simulink model "BMS2"  (R2024a)
settings: Solver=VariableStepAuto  StartTime=0.0  StopTime=3600  RelTol=1e-3
undefined symbols (not defined in the file): Ion, Lithium
libraries: spsMosfetLib x9, spsSeriesRLCBranchLib x9, spsBatteryLib x8, spsVoltageMeasurementLib x1, spsControlledCurrentSourceLib x1, spsDCVoltageSourceLib x1, spsDiodeLib x1, spsIdealSwitchLib x1, sps_lib x1
settings Model: Creator=kanna  LastModifiedBy=kanna

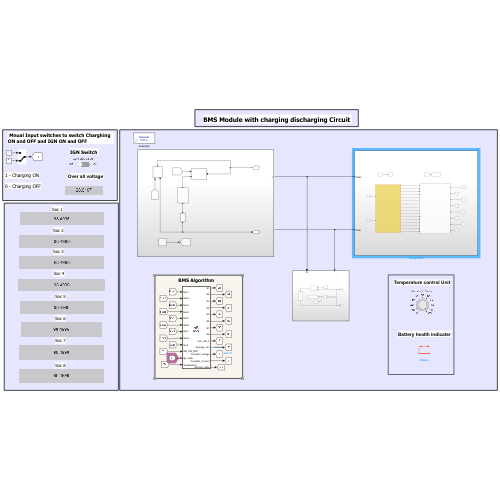
[thumbnail: Simulink's stored preview of the top-level diagram]
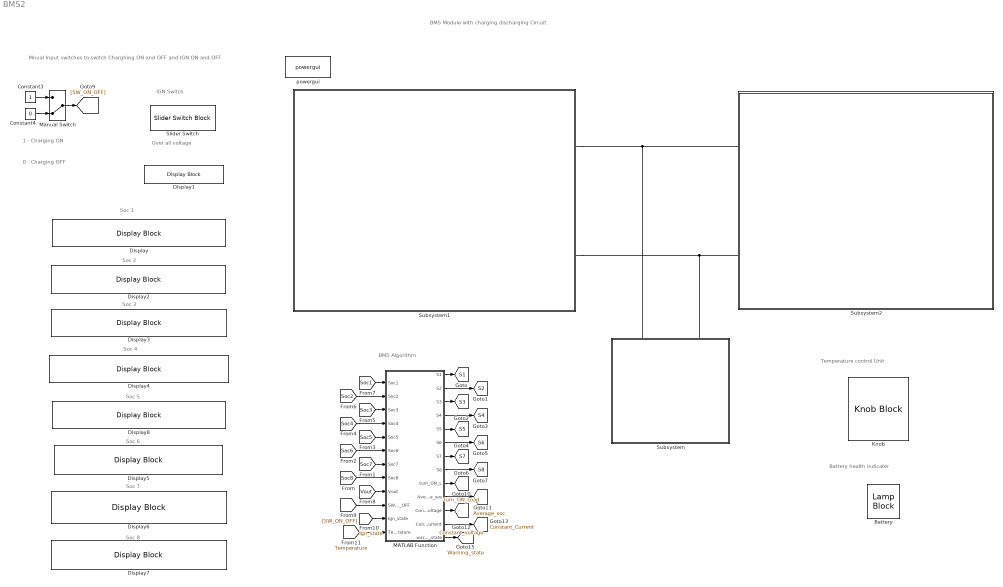
== system BMS2 ==
  note: Over all voltage
  note: Battery health indicater
  note: Temperature control Unit
  note: IGN Switch
  note: Soc 1
  note: 0 - Charging OFF
  note: 1 - Charging ON
  note: Mnual Input switches to switch Charghing ON and OFF and IGN ON and OFF
  note: BMS Algorithm
  note: BMS Module with charging discharging Circuit
  note: Soc 2
  note: Soc 3
  note: Soc 4
  note: Soc 5
  note: Soc 6
  note: Soc 7
  note: Soc 8
  Battery : LampBlock  LabelPosition=Hide  Icon=Battery
  Constant3 : Constant
  Constant4 : Constant  Value=0
  Display{,1..8} (9 alike) : DisplayBlock  LabelPosition=Hide  Transparency=1
  Knob : KnobBlock
  MATLAB Function : MATLAB Function  TreatAsAtomicUnit=on
  Manual Switch : ManualSwitch  CurrentSetting=0
  Slider Switch : SliderSwitchBlock
      settings: Values={{'Off', 'On'}, [0 1]}
  Subsystem : Subsystem
  Subsystem1 : Subsystem
  Subsystem2 : Subsystem
  powergui : sps_lib/powergui  Priority=1  SimulationMode=Discrete  SampleTime=10000e-6  frequency=60  Iterations=50  frequencyindice=0  Pbase=100e6  ErrMax=1e-4  UnitsV=kV  UnitsW=MW  buscounter=0  FunctionMessages=off  echomessages=off  EnableUseOfTLC=off  CurrentSourceSwitches=off  DisableSnubberDevices=off  DisableRonSwitches=off  DisableVfSwitches=off  DisplayEquations=off  AutomaticDiscreteSolvers=off  SolverType=Tustin/Backward Euler (TBE)  Interpol=off  ExternalGateDelay=off  methode=off  Ts=100  x0status=blocks  SPID=on  SwTol=0  HookPort=off  NonlinearTolerance=1e-4  nMaxIteration=100  ContinueOnMaxIteration=off  RestoreLinks=warning  ResistiveCurrentMeasurement=off  Frange=[0:2:500]  Ylog=off  Xlog=on  ShowGrid=off  save=off  variable=ZData  structure=0  ZoomFFT=off  StartTime=0.0  cycles=1  DisplayStyle=1  fundamental=60  FreqAxis=off  MaxFrequency=1000  frequencyindicesteady=1  RmsSteady=1  display=off
  tag scope: Average_soc=global, Constant_Current=global, Constant_voltage=global, S1=global, S2=global, S3=global, S4=global, S5=global, S6=global, S7=global, S8=global, Warning_state=global, turn_ON_Load=global
  wires:
  [Soc1] -> MATLAB Function/1(Soc1)
  [Soc2] -> MATLAB Function/2(Soc2)
  [Soc3] -> MATLAB Function/3(Soc3)
  [Soc4] -> MATLAB Function/4(Soc4)
  [Soc5] -> MATLAB Function/5(Soc5)
  [Soc6] -> MATLAB Function/6(Soc6)
  [Soc7] -> MATLAB Function/7(Soc7)
  [Soc8] -> MATLAB Function/8(Soc8)
  MATLAB Function/1(S1) -> [S1]
  MATLAB Function/5(S5) -> [S5]
  MATLAB Function/2(S2) -> [S2]
  MATLAB Function/3(S3) -> [S3]
  MATLAB Function/4(S4) -> [S4]
  MATLAB Function/6(S6) -> [S6]
  MATLAB Function/7(S7) -> [S7]
  MATLAB Function/8(S8) -> [S8]
  [Vout] -> MATLAB Function/9(Vout)
  Constant3/1 -> Manual Switch/1
  Constant4/1 -> Manual Switch/2
  Manual Switch/1 -> [SW_ON_OFF]
  [SW_ON_OFF] -> MATLAB Function/10(SW_ON_OFF)
  MATLAB Function/9(turn_ON_L) -> [turn_ON_Load]
  MATLAB Function/10(Average_soc) -> [Average_soc]
  MATLAB Function/11(Constant_voltage) -> [Constant_voltage]
  MATLAB Function/12(Constant_Current) -> [Constant_Current]
  [Ign_state] -> MATLAB Function/11(Ign_state)
  [Temperature] -> MATLAB Function/12(Temperature)
  MATLAB Function/13(warning_state) -> [Warning_state]
  connections:
  Subsystem1/RConn1 -- Subsystem2/LConn1 -- Subsystem/LConn1
  Subsystem1/RConn2 -- Subsystem2/LConn2 -- Subsystem/LConn2

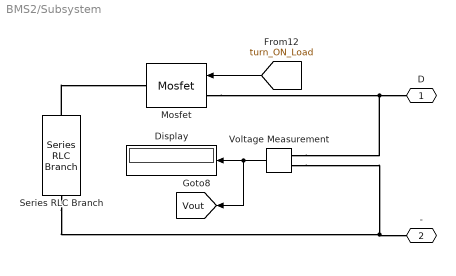
== system BMS2/Subsystem ==
  Display : Display
  Mosfet : spsMosfetLib/Mosfet  Ron=0.1  Lon=0  Rd=0.01  Vfd=0  IC=0  Rs=1e5  Cs=inf  Measurements=off
  Series RLC Branch : spsSeriesRLCBranchLib/Series RLC Branch  LConnTagsString=__new0  RConnTagsString=__new0  BranchType=R  Resistance=50  Inductance=1e-3  SetiL0=off  InitialCurrent=0  Capacitance=1e-6  Setx0=off  InitialVoltage=0  Measurements=None
  Voltage Measurement : spsVoltageMeasurementLib/Voltage Measurement  PhasorSimulation=off  OutputType=Complex  PSBequivalent=0
  D : PMIOPort  Side=Left
  - : PMIOPort  Port=2  Side=Left
  tag scope: Vout=global
  wires:
  [turn_ON_Load] -> Mosfet/1
  Voltage Measurement/1 -> [Vout], Display/1
  connections:
  Series RLC Branch/LConn1 -- Mosfet/RConn1
  Voltage Measurement/LConn1 -- Mosfet/LConn1 -- D/RConn1
  Series RLC Branch/RConn1 -- Voltage Measurement/LConn2 -- -/RConn1

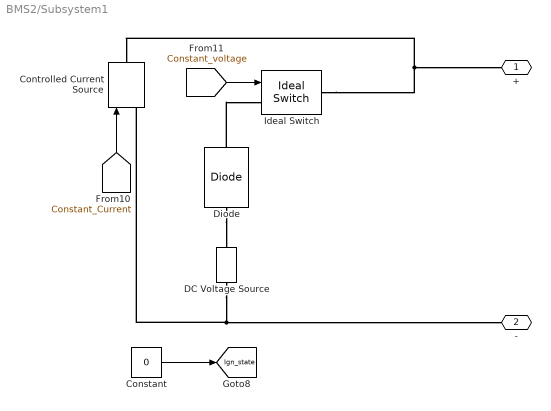
== system BMS2/Subsystem1 ==
  Constant : Constant  Value=0
  Controlled Current Source : spsControlledCurrentSourceLib/Controlled Current Source  Initialize=on  Source_Type=DC  Amplitude=2  Phase=0  Frequency=0  Measurements=None
  DC Voltage Source : spsDCVoltageSourceLib/DC Voltage Source  Amplitude=35  Measurements=None
  Diode : spsDiodeLib/Diode  Ron=0.001  Lon=0  Vf=0.8  IC=0  UseSnubber=0  Rs=500  Cs=250e-9  Measurements=off
  Ideal Switch : spsIdealSwitchLib/Ideal Switch  Ron=0.001  Lon=0  IC=0  Rs=1e5  Cs=inf  Measurements=off
  + : PMIOPort  Side=Right
  - : PMIOPort  Port=2  Side=Right
  tag scope: Ign_state=global
  wires:
  [Constant_voltage] -> Ideal Switch/1
  [Constant_Current] -> Controlled Current Source/1
  Constant/1 -> [Ign_state]
  connections:
  Ideal Switch/RConn1 -- +/RConn1 -- Controlled Current Source/RConn1
  Diode/RConn1 -- Ideal Switch/LConn1
  Diode/LConn1 -- DC Voltage Source/RConn1
  DC Voltage Source/LConn1 -- -/RConn1 -- Controlled Current Source/LConn1

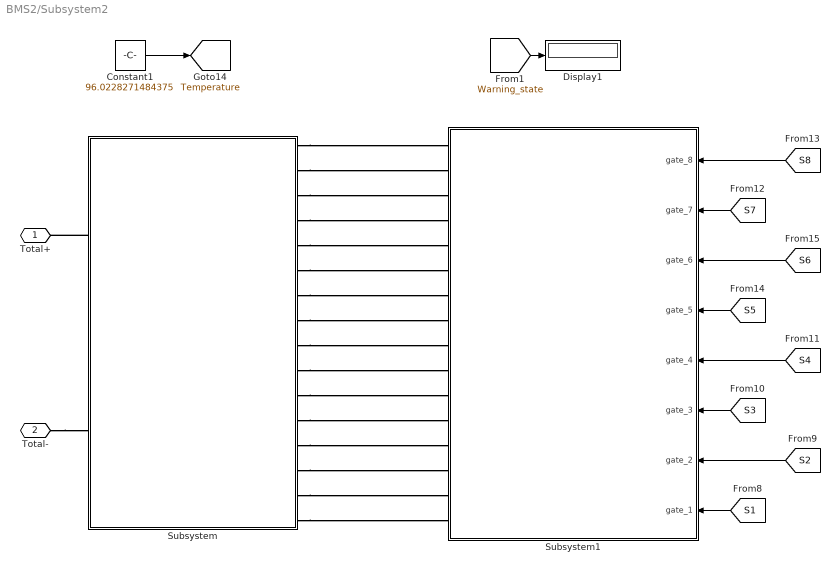
== system BMS2/Subsystem2 ==
  Constant1 : Constant  Value=96.0228271484375
  Display1 : Display
  Subsystem : Subsystem
  Subsystem1 : Subsystem
      settings: PortSchema="{\"entries\":[{\"content\":{\"sides\":[{\"content\":{\"connectorIds\":[\"LConn1\",\"LConn2\",\"LConn3\",\"LConn4\",\"LConn5\",\"LConn6\",\"LConn7\",\"LConn8\",\"LConn9\",\"LConn10\",\"LConn11\",\"LConn12\",\"LConn13\",\"LConn14\",\"LConn15\",\"LConn16\"]},\"type\":\"ConnectorPlacement.EquallySpacedRectSide\",\"uuid\":\"299ba52d-8015-465c-9de8-ad4a2af20b1b\"},{\"content\":{\"connectorIds\":[\"In1\",\"In2\",\"In3\",\"In4\",\"In5\",\"In6\",\"In7\",\"In8\"],\"side\":\"RIGHT\"},\"type\":\"ConnectorPlacement.EquallySpacedRectSide\",\"uuid\":\"0c259d42-c7d5-4490-aca3-04d7e6d01d9f\"},{\"content\":{\"side\":\"TOP\"},\"type\":\"ConnectorPlacement.EquallySpacedRectSide\",\"uuid\":\"1f9aba9e-79c3-4f87-9285-0c028554fb61\"}]},\"type\":\"ConnectorPlacement.EquallySpacedConnector\",\"uuid\":\"3efdec2a-ca98-432c-aa70-a3544e884ae7\"}],\"packageUris\":[\"http://schema.mathworks.com/mf0/Connector/R2020b\"],\"version\":\"1.0\"}"
  Total+ : PMIOPort  Side=Left
  Total- : PMIOPort  Port=2  Side=Left
  tag scope: Temperature=global
  wires:
  [S1] -> Subsystem1/8(gate_1)
  [S4] -> Subsystem1/5(gate_4)
  [S8] -> Subsystem1/1(gate_8)
  [S3] -> Subsystem1/6(gate_3)
  [S7] -> Subsystem1/2(gate_7)
  [S6] -> Subsystem1/3(gate_6)
  [S5] -> Subsystem1/4(gate_5)
  [S2] -> Subsystem1/7(gate_2)
  [Warning_state] -> Display1/1
  Constant1/1 -> [Temperature]
  connections:
  Subsystem/RConn11 -- Subsystem1/LConn11
  Subsystem/RConn2 -- Subsystem1/LConn2
  Subsystem/RConn8 -- Subsystem1/LConn8
  Subsystem/RConn9 -- Subsystem1/LConn9
  Subsystem/RConn5 -- Subsystem1/LConn5
  Total-/RConn1 -- Subsystem/LConn2
  Subsystem/LConn1 -- Total+/RConn1
  Subsystem/RConn3 -- Subsystem1/LConn3
  Subsystem/RConn7 -- Subsystem1/LConn7
  Subsystem/RConn4 -- Subsystem1/LConn4
  Subsystem/RConn1 -- Subsystem1/LConn1
  Subsystem/RConn16 -- Subsystem1/LConn16
  Subsystem/RConn6 -- Subsystem1/LConn6
  Subsystem/RConn12 -- Subsystem1/LConn12
  Subsystem/RConn14 -- Subsystem1/LConn14
  Subsystem/RConn10 -- Subsystem1/LConn10
  Subsystem/RConn13 -- Subsystem1/LConn13
  Subsystem/RConn15 -- Subsystem1/LConn15

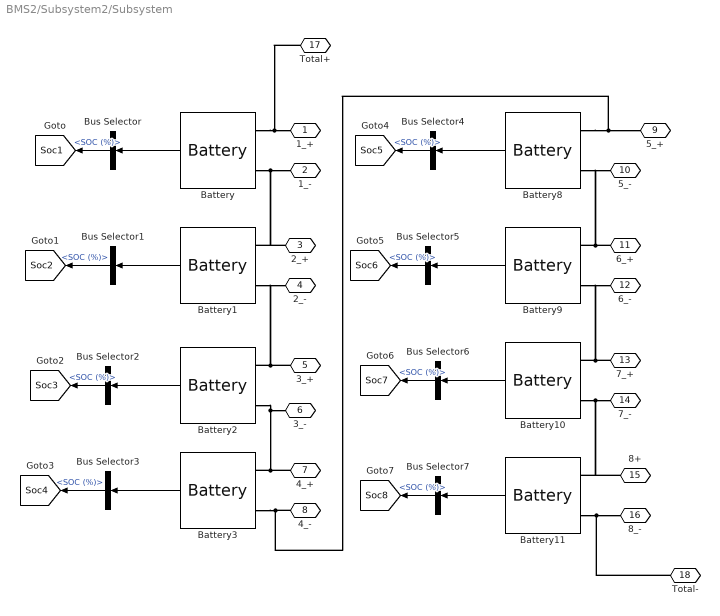
== system BMS2/Subsystem2/Subsystem ==
  Battery : spsBatteryLib/Battery  BatType=Lithium-Ion  ShowTempParam=off  ThermalPreset=no  ShowAgeParam=off  NomV=3.2  NomQ=18  SOC=98.5  Batt_Tr=30  PresetModel=on  MaxQ=18  MinV=2.4  FullV=3.7248  Dis_rate=7.8261  R=0.0017778  Normal_OP=16.2783  expZone="[3.4572     0.88435]"  current=[6.5 13 32.5]  Units=Time  Tci=20  NomT=20  T2=-30  MaxQ2=4.8  FullV2=7.1  Normal_OP2=5.655  expZone2="[6.58           1]"  Rca=0.6  ti=2000  Dp=0  Neq0=0  Tsim=1e6  Ta1=25  Qeol=5.4*0.9  Reol=0.013333*1.2  Char_age=[2.3478, 3]  Dis_age=[2.3478, 10]  N1=1500  N2=10500  N3=1000  N4=1400  Ta2=45  N5=950
  Battery1 : spsBatteryLib/Battery  BatType=Lithium-Ion  ShowTempParam=off  ThermalPreset=no  ShowAgeParam=off  NomV=3.2  NomQ=18  SOC=99  Batt_Tr=30  PresetModel=on  MaxQ=18  MinV=2.4  FullV=3.7248  Dis_rate=7.8261  R=0.0017778  Normal_OP=16.2783  expZone="[3.4572     0.88435]"  current=[6.5 13 32.5]  Units=Time  Tci=20  NomT=20  T2=-30  MaxQ2=4.8  FullV2=7.1  Normal_OP2=5.655  expZone2="[6.58           1]"  Rca=0.6  ti=2000  Dp=0  Neq0=0  Tsim=1e6  Ta1=25  Qeol=5.4*0.9  Reol=0.013333*1.2  Char_age=[2.3478, 3]  Dis_age=[2.3478, 10]  N1=1500  N2=10500  N3=1000  N4=1400  Ta2=45  N5=950
  Battery{2..3,8..11} (6 alike) : spsBatteryLib/Battery  BatType=Lithium-Ion  ShowTempParam=off  ThermalPreset=no  ShowAgeParam=off  NomV=3.2  NomQ=18  SOC=100  Batt_Tr=30  PresetModel=on  MaxQ=18  MinV=2.4  FullV=3.7248  Dis_rate=7.8261  R=0.0017778  Normal_OP=16.2783  expZone="[3.4572     0.88435]"  current=[6.5 13 32.5]  Units=Time  Tci=20  NomT=20  T2=-30  MaxQ2=4.8  FullV2=7.1  Normal_OP2=5.655  expZone2="[6.58           1]"  Rca=0.6  ti=2000  Dp=0  Neq0=0  Tsim=1e6  Ta1=25  Qeol=5.4*0.9  Reol=0.013333*1.2  Char_age=[2.3478, 3]  Dis_age=[2.3478, 10]  N1=1500  N2=10500  N3=1000  N4=1400  Ta2=45  N5=950
  Bus Selector{,1..7} (8 alike) : BusSelector  OutputSignals=SOC (%)
  1_+ : PMIOPort  Side=Right
  1_- : PMIOPort  Port=2  Side=Right
  2_+ : PMIOPort  Port=3  Side=Right
  2_- : PMIOPort  Port=4  Side=Right
  3_+ : PMIOPort  Port=5  Side=Right
  3_- : PMIOPort  Port=6  Side=Right
  4_+ : PMIOPort  Port=7  Side=Right
  4_- : PMIOPort  Port=8  Side=Right
  5_+ : PMIOPort  Port=9  Side=Right
  5_- : PMIOPort  Port=10  Side=Right
  6_+ : PMIOPort  Port=11  Side=Right
  6_- : PMIOPort  Port=12  Side=Right
  7_+ : PMIOPort  Port=13  Side=Right
  7_- : PMIOPort  Port=14  Side=Right
  8+ : PMIOPort  Port=15  Side=Right
  8_- : PMIOPort  Port=16  Side=Right
  Total+ : PMIOPort  Port=17  Side=Left
  Total- : PMIOPort  Port=18  Side=Left
  tag scope: Soc1=global, Soc2=global, Soc3=global, Soc4=global, Soc5=global, Soc6=global, Soc7=global, Soc8=global
  wires:
  Battery1/1 -> Bus Selector1/1
  Bus Selector/1 -> [Soc1]  "<SOC (%)>"
  Battery/1 -> Bus Selector/1
  Bus Selector7/1 -> [Soc8]  "<SOC (%)>"
  Bus Selector5/1 -> [Soc6]  "<SOC (%)>"
  Battery2/1 -> Bus Selector2/1
  Battery11/1 -> Bus Selector7/1
  Bus Selector4/1 -> [Soc5]  "<SOC (%)>"
  Bus Selector6/1 -> [Soc7]  "<SOC (%)>"
  Battery3/1 -> Bus Selector3/1
  Bus Selector3/1 -> [Soc4]  "<SOC (%)>"
  Bus Selector2/1 -> [Soc3]  "<SOC (%)>"
  Bus Selector1/1 -> [Soc2]  "<SOC (%)>"
  Battery8/1 -> Bus Selector4/1
  Battery10/1 -> Bus Selector6/1
  Battery9/1 -> Bus Selector5/1
  connections:
  Battery11/LConn2 -- 8_-/RConn1 -- Total-/RConn1
  3_+/RConn1 -- Battery2/LConn1 -- Battery1/LConn2 -- 2_-/RConn1
  3_-/RConn1 -- Battery2/LConn2 -- 4_+/RConn1 -- Battery3/LConn1
  7_+/RConn1 -- Battery10/LConn1 -- Battery9/LConn2 -- 6_-/RConn1
  Battery10/LConn2 -- 7_-/RConn1 -- 8+/RConn1 -- Battery11/LConn1
  Battery/LConn2 -- 1_-/RConn1 -- 2_+/RConn1 -- Battery1/LConn1
  Total+/RConn1 -- Battery/LConn1 -- 1_+/RConn1
  6_+/RConn1 -- Battery9/LConn1 -- Battery8/LConn2 -- 5_-/RConn1
  Battery8/LConn1 -- 4_-/RConn1 -- Battery3/LConn2 -- 5_+/RConn1

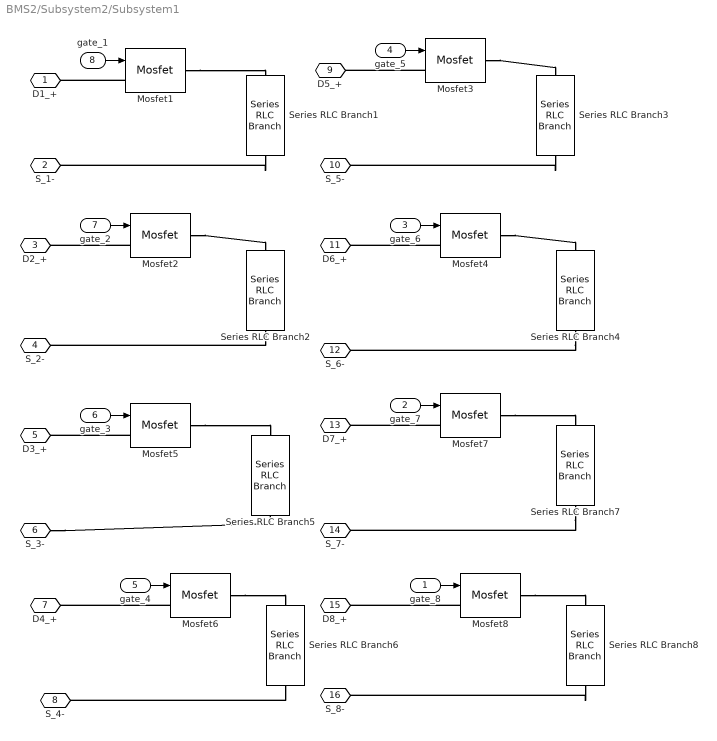
== system BMS2/Subsystem2/Subsystem1 ==
  gate_8 : Inport
  gate_7 : Inport  Port=2
  gate_6 : Inport  Port=3
  gate_5 : Inport  Port=4
  gate_4 : Inport  Port=5
  gate_3 : Inport  Port=6
  gate_2 : Inport  Port=7
  gate_1 : Inport  Port=8
  Mosfet{1..8} (8 alike) : spsMosfetLib/Mosfet  Ron=0.1  Lon=0  Rd=0.01  Vfd=0  IC=0  Rs=1e5  Cs=inf  Measurements=off
  Series RLC Branch{1..8} (8 alike) : spsSeriesRLCBranchLib/Series RLC Branch  LConnTagsString=__new0  RConnTagsString=__new0  BranchType=R  Resistance=1  Inductance=1e-3  SetiL0=off  InitialCurrent=0  Capacitance=1e-6  Setx0=off  InitialVoltage=0  Measurements=None
  D1_+ : PMIOPort  Side=Left
  S_1- : PMIOPort  Port=2  Side=Left
  D2_+ : PMIOPort  Port=3  Side=Left
  S_2- : PMIOPort  Port=4  Side=Left
  D3_+ : PMIOPort  Port=5  Side=Left
  S_3- : PMIOPort  Port=6  Side=Left
  D4_+ : PMIOPort  Port=7  Side=Left
  S_4- : PMIOPort  Port=8  Side=Left
  D5_+ : PMIOPort  Port=9  Side=Left
  S_5- : PMIOPort  Port=10  Side=Left
  D6_+ : PMIOPort  Port=11  Side=Left
  S_6- : PMIOPort  Port=12  Side=Left
  D7_+ : PMIOPort  Port=13  Side=Left
  S_7- : PMIOPort  Port=14  Side=Left
  D8_+ : PMIOPort  Port=15  Side=Left
  S_8- : PMIOPort  Port=16  Side=Left
  wires:
  gate_1/1 -> Mosfet1/1
  gate_6/1 -> Mosfet4/1
  gate_2/1 -> Mosfet2/1
  gate_3/1 -> Mosfet5/1
  gate_7/1 -> Mosfet7/1
  gate_8/1 -> Mosfet8/1
  gate_5/1 -> Mosfet3/1
  gate_4/1 -> Mosfet6/1
  connections:
  Mosfet2/RConn1 -- Series RLC Branch2/LConn1
  Mosfet8/RConn1 -- Series RLC Branch8/LConn1
  Mosfet4/RConn1 -- Series RLC Branch4/LConn1
  Mosfet6/RConn1 -- Series RLC Branch6/LConn1
  Mosfet1/RConn1 -- Series RLC Branch1/LConn1
  Mosfet3/RConn1 -- Series RLC Branch3/LConn1
  Mosfet5/RConn1 -- Series RLC Branch5/LConn1
  Mosfet2/LConn1 -- D2_+/RConn1
  Mosfet7/RConn1 -- Series RLC Branch7/LConn1
  Mosfet6/LConn1 -- D4_+/RConn1
  Series RLC Branch2/RConn1 -- S_2-/RConn1
  Series RLC Branch4/RConn1 -- S_6-/RConn1
  Mosfet4/LConn1 -- D6_+/RConn1
  Series RLC Branch8/RConn1 -- S_8-/RConn1
  Mosfet8/LConn1 -- D8_+/RConn1
  Mosfet7/LConn1 -- D7_+/RConn1
  Series RLC Branch6/RConn1 -- S_4-/RConn1
  Mosfet5/LConn1 -- D3_+/RConn1
  Series RLC Branch7/RConn1 -- S_7-/RConn1
  Series RLC Branch1/RConn1 -- S_1-/RConn1
  S_3-/RConn1 -- Series RLC Branch5/RConn1
  Series RLC Branch3/RConn1 -- S_5-/RConn1
  Mosfet3/LConn1 -- D5_+/RConn1
  Mosfet1/LConn1 -- D1_+/RConn1

== matlab function BMS2/MATLAB Function ==
  data: Soc1 input; S1 output; Soc2 input; Soc3 input; Soc4 input; Soc5 input; Soc6 input; Soc7 input; Soc8 input; S2 output; S3 output; S4 output; S5 output; S6 output; S7 output; S8 output; Vout input; SW_ON_OFF input; turn_ON_L output; Average_soc output; Constant_voltage output; Constant_Current output; Ign_state input; Temperature input; warning_state output
function [S1, S2, S3, S4, S5, S6, S7, S8, turn_ON_L, Average_soc, Constant_voltage, Constant_Current,warning_state] = BMS(Soc1, Soc2, Soc3, Soc4, Soc5, Soc6, Soc7, Soc8, Vout, SW_ON_OFF,Ign_state, Temperature)
    [Constant_voltage, Constant_Current,turn_ON_L,Average_soc,warning_state] = deal(0); % Default value
    soc =int32([Soc1, Soc2, Soc3, Soc4, Soc5, Soc6, Soc7, Soc8]);
    [S1, S2, S3, S4, S5, S6, S7, S8] = deal(0);
    Same_soc= unique(soc);
 
    if isscalar(Same_soc)
     % Average Soc function
    Average_soc = Avg_soc(Soc1, Soc2, Soc3, Soc4, Soc5, Soc6, Soc7, Soc8);

    % Call operatingvolt function
    V_operating = operatingvolt(Vout);

    % Call Chargingvolt function
    charging = Chargingvolt(SW_ON_OFF);

    % To turn ON current or Voltage source
    if (Average_soc > 80 && Average_soc <= 100)&& charging
        Constant_voltage = 1;
        Constant_Current = 0;
    elseif Average_soc <= 80 && charging
        Constant_Current = 1;
        Constant_voltage = 0;
    end

    % To turn ON or OFF load
    if V_operating && (~charging) && Ign_state
        turn_ON_L = 1;
    else
        turn_ON_L = 0;
    end

    % to display warning when temperature exceeds safe operating limits 
    if (Temperature > 50 )&& (Temperature < 80)
        warning_state=1;
    elseif Temperature > 80
        warning_state =2;
    end

    % Display the results
    disp('turn_ON_L:');
    disp(turn_ON_L);
    disp('Average_soc:');
    disp(Average_soc);
    disp('Constant_voltage:');
    disp(Constant_voltage);
    disp('Constant_Current:');
    disp(Constant_Current);  
    disp('V_operating:');
    disp(V_operating);
    disp('charging:');
    disp(charging);
  
    else
      % Call Cell_balencing function
    
 
    [S1, S2, S3, S4, S5, S6, S7, S8 ]= cellbalencing (Soc1, Soc2, Soc3, Soc4, Soc5, Soc6, Soc7,Soc8);
    end
end

function V_operating = operatingvolt(Vout)
    V_max = 30;
    V_min = 22;
    Vout = int16(Vout);
    if Vout < V_max && Vout > V_min
        V_operating = 1;
    else
        V_operating = 0;
    end
end

function charging = Chargingvolt(SW_ON_OFF)
    if SW_ON_OFF == 1
        charging = 1;
    else
        charging = 0;
    end
end

function Average_soc = Avg_soc(Soc1, Soc2, Soc3, Soc4, Soc5, Soc6, Soc7, Soc8)
    Avg_soc = [Soc1, Soc2, Soc3, Soc4, Soc5, Soc6, Soc7, Soc8];
    Average_soc = mean(Avg_soc);
end

function [S1, S2, S3, S4, S5, S6, S7, S8] = cellbalencing (Soc1, Soc2, Soc3, Soc4, Soc5, Soc6, Soc7,Soc8)
    SocArray = int32([Soc1, Soc2, Soc3, Soc4, Soc5, Soc6, Soc7, Soc8]);
    


    % Initialize Switch array
    Switch_sel = zeros(1,8);

    % Find the minimum SoC
    min_soc = min(SocArray);
   
    

    % Perform cell balancing

  
       
   
    for i = 1:length(SocArray)
        if SocArray(i) > min_soc
            Switch_sel(i) = 1;
        elseif SocArray(i) <= min_soc
            Switch_sel(i) = 0;
        end
 

    % Assign outputs
 S1= Switch_sel(1);
 S2= Switch_sel(2);
 S3= Switch_sel(3);
 S4= Switch_sel(4);
 S5= Switch_sel(5);
 S6= Switch_sel(6);
 S7= Switch_sel(7);
 S8= Switch_sel(8);

    end
   end
